simulink model "TD2"  (Simulink 9.0)
settings: Solver=VariableStepAuto  StartTime=0.0  StopTime=10.0  RelTol=1e-3
InitFcn:
  | TD2_config
StartFcn:
  | TD2_config
values from neighbouring files (symbols this model uses):
  b = 8.5E-3    (= 0.0085)    [TD2_config.m]
  J = 0.28    [TD2_config.m]
  K = 0.5093    [TD2_config.m]
  Kd = 0    [TD2_config.m]
  Ki = 0    [TD2_config.m]
  Kp = 0    [TD2_config.m]
  L = 1.6E-3    (= 0.0016)    [TD2_config.m]
  R = 0.13    [TD2_config.m]
settings Model: Creator=TABLE 6  LastModifiedBy=TABLE 6
settings DataIOCC: SaveFormat=Dataset
settings OptimizationCC: LifeSpan=auto
settings DebuggingCC: UnderspecifiedInitializationDetection=Simplified  MergeDetectMultiDrivingBlocksExec=error  SFUnexpectedBacktrackingDiag=error  SFNoUnconditionalDefaultTransitionDiag=error  SFExecutionAtInitializationDiag=warning
settings HardwareCC: ProdBitPerPointer=64  ProdBitPerSizeT=64  ProdBitPerPtrDiffT=64  ProdLargestAtomicFloat=Float  ProdIntDivRoundTo=Zero  ProdEndianess=LittleEndian  ProdWordSize=64  ProdHWDeviceType=Intel->x86-64 (Windows64)
settings ModelReferenceCC: PropagateSignalLabelsOutOfModel=on
settings CodeAppCC: StateflowObjectComments=off
settings GRTTargetCC: TargetLangStandard=C99 (ISO)
settings ConfigComp: CovMetricSettings=dwe  CovHtmlReporting=off  CovSaveCumulativeToWorkspaceVar=off  CovSaveSingleToWorkspaceVar=off  CovExternalEMLEnable=on

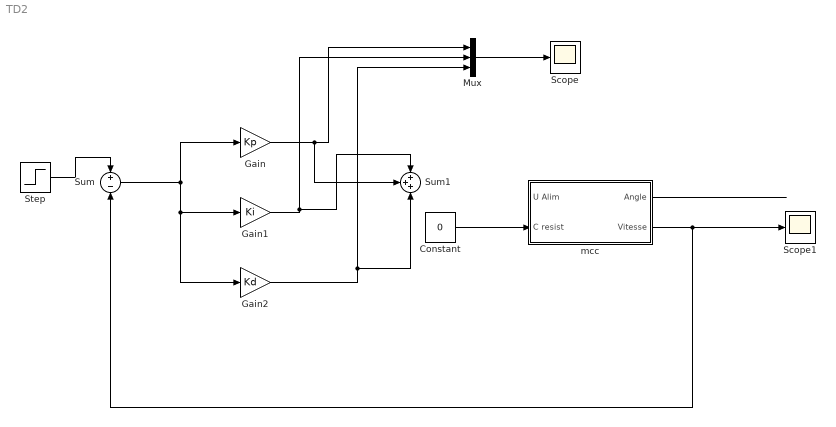
== system TD2 ==
  Constant : Constant  Value=0
  Gain : Gain  Gain=Kp
  Gain1 : Gain  Gain=Ki
  Gain2 : Gain  Gain=Kd
  Mux : Mux  Inputs=3
  Scope : Scope
  Scope1 : Scope
  Step : Step  Time=0  SampleTime=0
  Sum : Sum  Inputs=+|-
  Sum1 : Sum  Inputs=+++
  mcc : Subsystem
  wires:
  Gain/1 -> Sum1/2, Mux/1
  Gain1/1 -> Sum1/1, Mux/2
  Gain2/1 -> Sum1/3, Mux/3
  Constant/1 -> mcc/2(C resist)
  Mux/1 -> Scope/1
  mcc/2(Vitesse) -> Sum/2, Scope1/1
  mcc/1(Angle) -> ?
  Step/1 -> Sum/1
  Sum/1 -> Gain2/1, Gain1/1, Gain/1

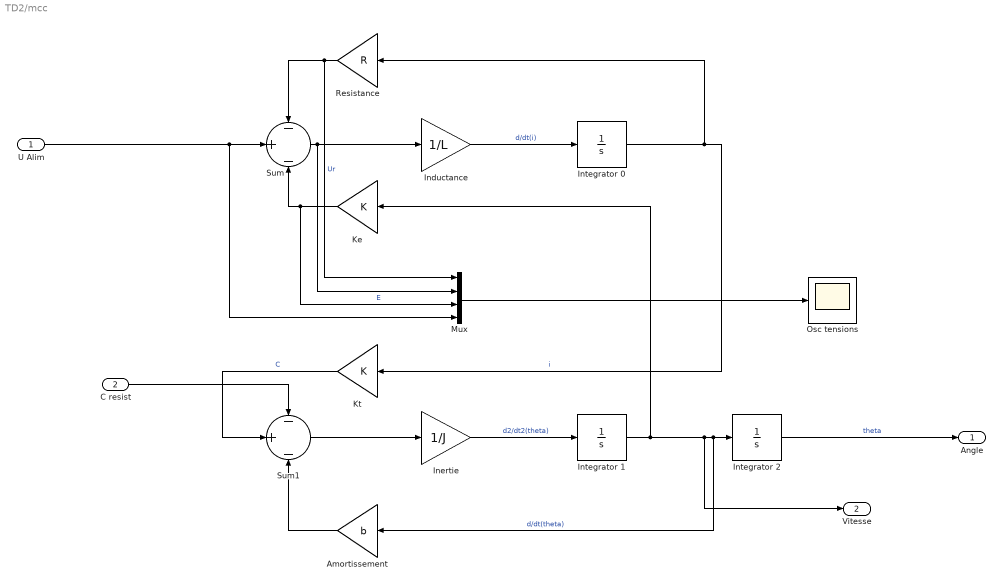
== system TD2/mcc ==
  U Alim : Inport
  C resist : Inport  Port=2
  "\tAmortissement" : Gain  Gain=b
  "\tInductance" : Gain  Gain=1/L
  "\tInertie" : Gain  Gain=1/J
  "\tKe" : Gain  Gain=K
  "\tKt" : Gain  Gain=K
  "\tResistance" : Gain  Gain=R
  Integrator 0 : Integrator
  "Integrator 1 " : Integrator
  "Integrator 2 " : Integrator
  Mux : Mux
  Osc tensions : Scope
  Sum : Sum  Inputs=-|+|-
  Sum1 : Sum  Inputs=-|+|-
  Angle : Outport
  Vitesse : Outport  Port=2
  wires:
  "Integrator 2 "/1 -> Angle/1  "theta"
  "\tResistance"/1 -> Mux/1, Sum/1  "Ur"
  C resist/1 -> Sum1/1
  Mux/1 -> Osc tensions/1
  "\tAmortissement"/1 -> Sum1/3
  "\tKe"/1 -> Mux/3, Sum/3  "E"
  "\tKt"/1 -> Sum1/2  "C"
  Integrator 0/1 -> "\tResistance"/1, "\tKt"/1  "i"
  "\tInertie"/1 -> "Integrator 1 "/1  "d2/dt2(theta)"
  Sum1/1 -> "\tInertie"/1
  U Alim/1 -> Mux/4, Sum/2
  "Integrator 1 "/1 -> "\tKe"/1, Vitesse/1, "\tAmortissement"/1, "Integrator 2 "/1  "d/dt(theta)"
  Sum/1 -> Mux/2, "\tInductance"/1
  "\tInductance"/1 -> Integrator 0/1  "d/dt(i)"
